simulink model "LevitadorMagnetico_act3"  (R2021a)
settings: Solver=ode1  StartTime=0.0  StopTime=1  FixedStep=0.001  RelTol=1e-3
settings Model: Creator=zeta  LastModifiedBy=zeta

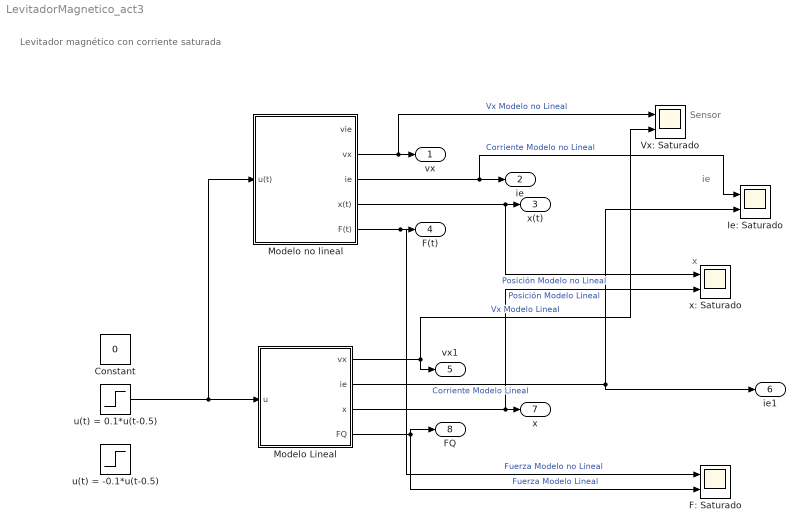
== system LevitadorMagnetico_act3 ==
  note: Levitador magnético con corriente saturada
  note: ie
  note: Sensor
  note: x
  Constant : Constant  Value=0
  F: Saturado : Scope  NumInputPorts=2
  Ie: Saturado : Scope  NumInputPorts=2
  Modelo Lineal : Subsystem  mask{Ka=3, Km=1, K1=5888, K2=1536, R=20, L=0.2, uQ=0, xQ=3.2, vxQ=3.2, ieQ=0, vx_sat_sup=0-3.2, vx_sat_inf=-10-3.2, x_sat_sup=10-3.2, x_sat_inf=-3.2, m=0.15, g=1000}
      mask prompts: vx_sat_sup "(vx_sat_sup - vxQ)"; vx_sat_inf "(vx_sat_inf- vxQ)"; x_sat_sup "(x_sat_sup - xQ)"; x_sat_inf "(x_sat_inf  - xQ)"
      mask DialogControl Control2 Prompt: Punto de operación:
      mask DialogControl Control3 Prompt: Saturación:
      mask DialogControl Control4 Prompt: otros
  Modelo no lineal : Subsystem
  Vx: Saturado : Scope  NumInputPorts=2
  u(t) = -0.1*u(t-0.5) : Step  Time=0.5  After=-0.1  SampleTime=0
  u(t) = 0.1*u(t-0.5) : Step  Time=0.5  After=0.1  SampleTime=0
  x: Saturado : Scope  NumInputPorts=2
  vx : Outport
  ie : Outport  Port=2
  x(t) : Outport  Port=3
  F(t) : Outport  Port=4
  vx1 : Outport  Port=5
  ie1 : Outport  Port=6
  x : Outport  Port=7
  FQ : Outport  Port=8
  wires:
  Modelo no lineal/2(vx) -> Vx: Saturado/1, vx/1  "Vx Modelo no Lineal"
  Modelo no lineal/4(x(t)) -> x: Saturado/1, x(t)/1  "Posición Modelo no Lineal"
  Modelo no lineal/5(F(t)) -> F: Saturado/1, F(t)/1  "Fuerza Modelo no Lineal"
  Modelo Lineal/4(FQ) -> F: Saturado/2, FQ/1  "Fuerza Modelo Lineal"
  Modelo Lineal/2(ie) -> ie1/1, Ie: Saturado/2  "Corriente Modelo Lineal"
  Modelo Lineal/1(vx) -> vx1/1, Vx: Saturado/2  "Vx Modelo Lineal"
  Modelo Lineal/3(x) -> x: Saturado/2, x/1  "Posición Modelo Lineal"
  Modelo no lineal/3(ie) -> Ie: Saturado/1, ie/1  "Corriente Modelo no Lineal"
  u(t) = 0.1*u(t-0.5)/1 -> Modelo no lineal/1(u(t)), Modelo Lineal/1(u)

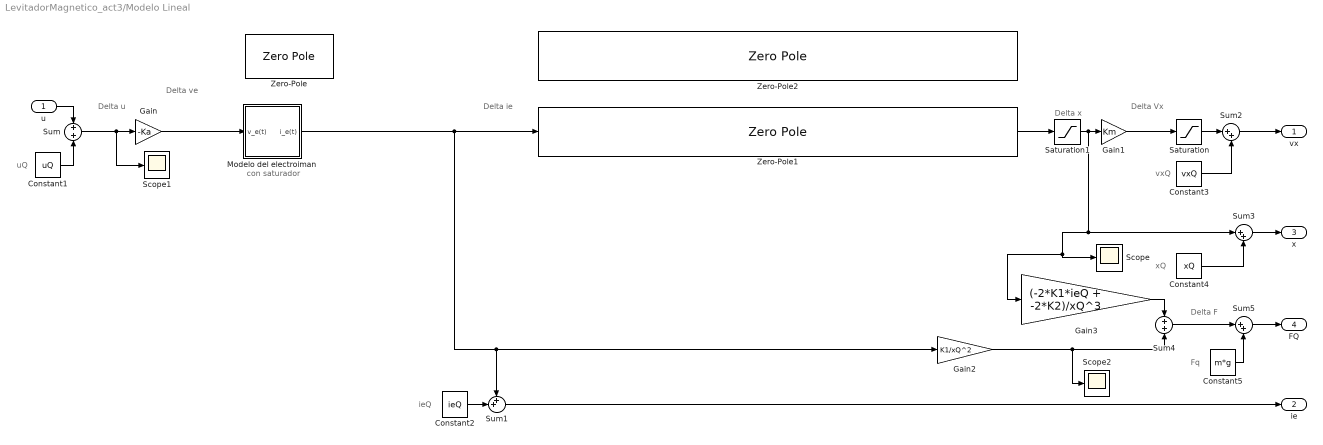
== system LevitadorMagnetico_act3/Modelo Lineal ==
  note: con saturador
  note: Fq
  note: Delta F
  note: vxQ
  note: Delta Vx
  note: Delta x
  note: Delta ie
  note: Delta ve
  note: Delta u
  note: uQ
  note: ieQ
  note: xQ
  u : Inport
  Constant1 : Constant  Value=uQ
  Constant2 : Constant  Value=ieQ
  Constant3 : Constant  Value=vxQ
  Constant4 : Constant  Value=xQ
  Constant5 : Constant  Value=m*g
  Gain : Gain  Gain=-Ka
  Gain1 : Gain  Gain=Km
  Gain2 : Gain  Gain=K1/xQ^2
  Gain3 : Gain  Gain=(-2*K1*ieQ + -2*K2)/xQ^3
  Modelo del electroiman : Subsystem  mask{L=0.2, R=20, ve_0=0}
      mask prompts: L "L [H]"; R "R [ohm]"; ve_0 "ve_0 [V]"
  Saturation : Saturate  UpperLimit=vx_sat_sup  LowerLimit=vx_sat_inf
  Saturation1 : Saturate  UpperLimit=x_sat_sup  LowerLimit=x_sat_inf
  Scope : Scope
  Scope1 : Scope
  Scope2 : Scope
  Sum : Sum  Inputs=+|+
  Sum1 : Sum  Inputs=++|
  Sum2 : Sum  Inputs=|++
  Sum3 : Sum  Inputs=|++
  Sum4 : Sum  Inputs=+|+
  Sum5 : Sum  Inputs=|++
  Zero-Pole : ZeroPole  Zeros=[]  Poles=[-R/L]  Gain=[1/L]
  Zero-Pole1 : ZeroPole  Zeros=[]  Poles=[-25 25]  Gain=[-K1/(m*xQ^2) ]
  Zero-Pole2 : ZeroPole  Zeros=[]  Poles=[-sqrt(2*(K1*ieQ + K2)/(m*xQ^3)) sqrt(2*(K1*ieQ + K2)/(m*xQ^3)) ]  Gain=[-K1/ (m*xQ^2) ]
  vx : Outport
  ie : Outport  Port=2
  x : Outport  Port=3
  FQ : Outport  Port=4
  wires:
  u/1 -> Sum/1
  Sum1/1 -> ie/1
  Sum3/1 -> x/1
  Constant2/1 -> Sum1/2
  Constant4/1 -> Sum3/2
  Sum2/1 -> vx/1
  Sum4/1 -> Sum5/1
  Gain1/1 -> Saturation/1
  Saturation/1 -> Sum2/1
  Zero-Pole1/1 -> Saturation1/1
  Constant5/1 -> Sum5/2
  Modelo del electroiman/1(i_e(t)) -> Zero-Pole1/1, Gain2/1, Sum1/1
  Saturation1/1 -> Gain1/1, Sum3/1, Scope/1, Gain3/1
  Sum5/1 -> FQ/1
  Constant1/1 -> Sum/2
  Sum/1 -> Scope1/1, Gain/1
  Constant3/1 -> Sum2/2
  Gain2/1 -> Scope2/1, Sum4/2
  Gain3/1 -> Sum4/1
  Gain/1 -> Modelo del electroiman/1(v_e(t))

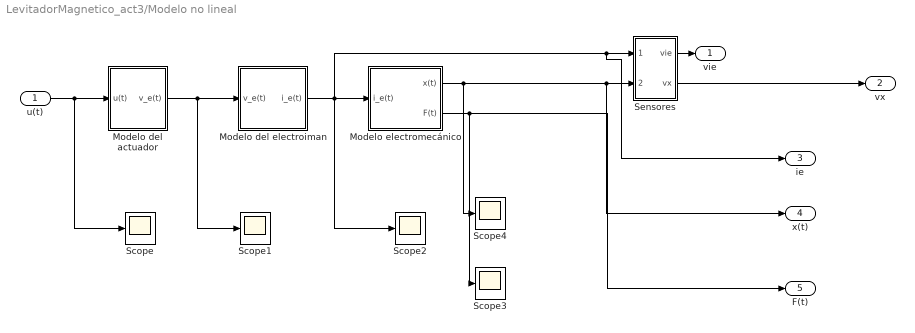
== system LevitadorMagnetico_act3/Modelo no lineal ==
  u(t) : Inport
  Modelo del actuador : Subsystem  mask{delta_a=0, K_a=3}
  Modelo del electroiman : Subsystem  mask{L=0.2, R=20, ve_0=0}
      mask prompts: L "L [H]"; R "R [ohm]"; ve_0 "ve_0 [V]"
  Modelo electromecánico : Subsystem  mask{K_1=5888, K_2=1536, m=0.15, g=1000, x0=3.2, v0=0}
  Scope{,1..4} (5 alike) : Scope
  Sensores : Subsystem  mask{delta_L=0, K_L=20/3, K_m=0, delta_m=10}
      mask prompts: K_m "1"
  vie : Outport
  vx : Outport  Port=2
  ie : Outport  Port=3
  x(t) : Outport  Port=4
  F(t) : Outport  Port=5
  wires:
  u(t)/1 -> Scope/1, Modelo del actuador/1(u(t))
  Modelo del actuador/1(v_e(t)) -> Scope1/1, Modelo del electroiman/1(v_e(t))
  Sensores/1(vie) -> vie/1
  Modelo del electroiman/1(i_e(t)) -> ie/1, Sensores/1(ie(t)), Modelo electromecánico/1(i_e(t)), Scope2/1
  Modelo electromecánico/1(x(t)) -> x(t)/1, Sensores/2(x(t)), Scope4/1
  Modelo electromecánico/2(F(t)) -> Scope3/1, F(t)/1
  Sensores/2(vx) -> vx/1

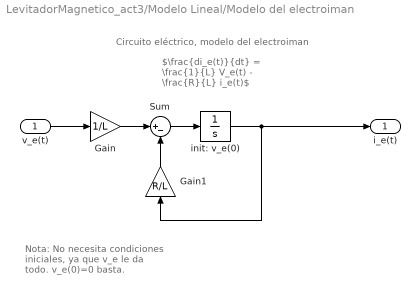
== system LevitadorMagnetico_act3/Modelo Lineal/Modelo del electroiman ==
  note: Nota: No necesita condiciones iniciales, ya que v_e le da todo.
      | v_e(0)=0 basta.
  note: $\frac{di_e(t)}{dt} = \frac{1}{L} V_e(t) - \frac{R}{L} i_e(t)$
  note: Circuito eléctrico, modelo del electroiman
  v_e(t) : Inport
  Gain : Gain  Gain=1/L
  Gain1 : Gain  Gain=R/L
  Sum : Sum  Inputs=|+-
  init: v_e(0) : Integrator  InitialCondition=ve_0  LimitOutput=on  UpperSaturationLimit=0.01  LowerSaturationLimit=-0.01
  i_e(t) : Outport
  wires:
  v_e(t)/1 -> Gain/1
  Gain/1 -> Sum/1
  init: v_e(0)/1 -> i_e(t)/1, Gain1/1
  Gain1/1 -> Sum/2
  Sum/1 -> init: v_e(0)/1

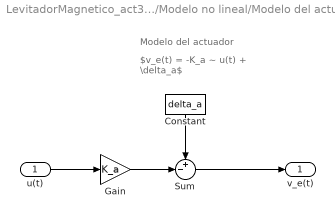
== system LevitadorMagnetico_act3/Modelo no lineal/Modelo del actuador ==
  note: $v_e(t) = -K_a ~ u(t) + \delta_a$
  note: Modelo del actuador
  u(t) : Inport
  Constant : Constant  Value=delta_a
  Gain : Gain  Gain=K_a
  Sum : Sum  Inputs=+-|
  v_e(t) : Outport
  wires:
  Constant/1 -> Sum/1
  Gain/1 -> Sum/2
  Sum/1 -> v_e(t)/1
  u(t)/1 -> Gain/1

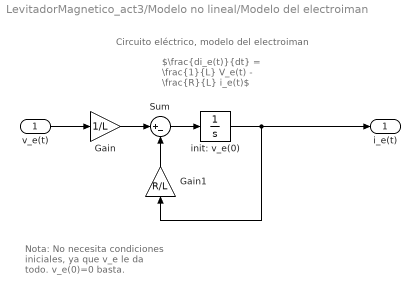
== system LevitadorMagnetico_act3/Modelo no lineal/Modelo del electroiman ==
  note: Nota: No necesita condiciones iniciales, ya que v_e le da todo.
      | v_e(0)=0 basta.
  note: $\frac{di_e(t)}{dt} = \frac{1}{L} V_e(t) - \frac{R}{L} i_e(t)$
  note: Circuito eléctrico, modelo del electroiman
  v_e(t) : Inport
  Gain : Gain  Gain=1/L
  Gain1 : Gain  Gain=R/L
  Sum : Sum  Inputs=|+-
  init: v_e(0) : Integrator  InitialCondition=ve_0  LimitOutput=on  UpperSaturationLimit=0.01  LowerSaturationLimit=-0.01
  i_e(t) : Outport
  wires:
  v_e(t)/1 -> Gain/1
  Gain/1 -> Sum/1
  init: v_e(0)/1 -> i_e(t)/1, Gain1/1
  Gain1/1 -> Sum/2
  Sum/1 -> init: v_e(0)/1

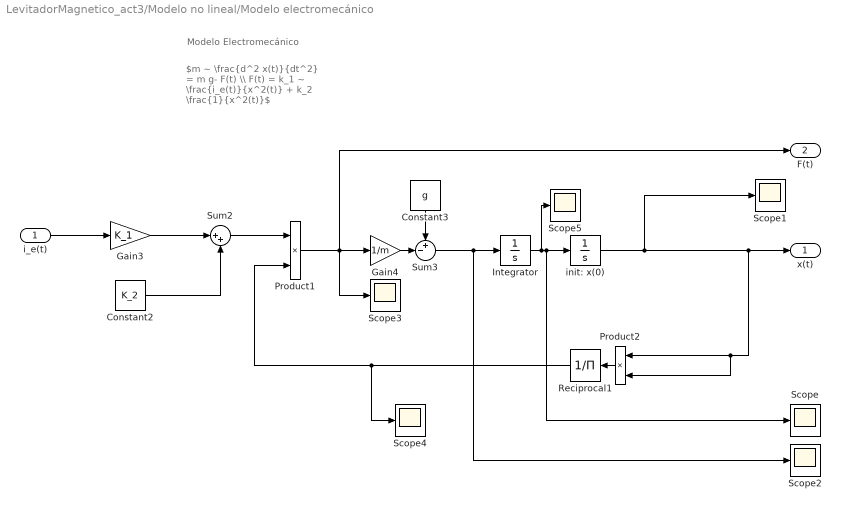
== system LevitadorMagnetico_act3/Modelo no lineal/Modelo electromecánico ==
  note: $m ~ \frac{d^2 x(t)}{dt^2} = m g- F(t) \\ F(t) = k_1 ~ \frac{i_e(t)}{x^2(t)} + k_2 \frac{1}{x^2(t)}$
  note: Modelo Electromecánico
  i_e(t) : Inport
  Constant2 : Constant  Value=K_2
  Constant3 : Constant  Value=g
  Gain3 : Gain  Gain=K_1
  Gain4 : Gain  Gain=1/m
  Integrator : Integrator  InitialCondition=v0  LowerSaturationLimit=0
  Product1 : Product
  Product2 : Product
  Reciprocal1 : Product  Inputs=/
  Scope{,1..5} (6 alike) : Scope
  Sum2 : Sum  Inputs=|++
  Sum3 : Sum  Inputs=+-|
  init: x(0) : Integrator  InitialCondition=x0  LimitOutput=on  UpperSaturationLimit=10  LowerSaturationLimit=1e-10
  x(t) : Outport
  F(t) : Outport  Port=2
  wires:
  i_e(t)/1 -> Gain3/1
  Gain3/1 -> Sum2/1
  Constant2/1 -> Sum2/2
  Sum2/1 -> Product1/1
  Constant3/1 -> Sum3/1
  Gain4/1 -> Sum3/2
  Sum3/1 -> Scope2/1, Integrator/1
  Product2/1 -> Reciprocal1/1
  init: x(0)/1 -> x(t)/1, Product2/1, Product2/2, Scope1/1
  Reciprocal1/1 -> Scope4/1, Product1/2
  Integrator/1 -> Scope5/1, init: x(0)/1, Scope/1
  Product1/1 -> Scope3/1, F(t)/1, Gain4/1

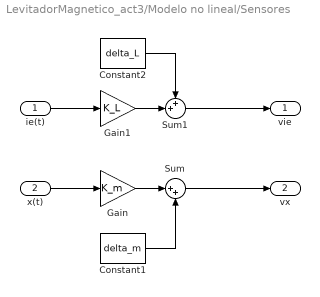
== system LevitadorMagnetico_act3/Modelo no lineal/Sensores ==
  ie(t) : Inport
  x(t) : Inport  Port=2
  Constant1 : Constant  Value=delta_m
  Constant2 : Constant  Value=delta_L
  Gain : Gain  Gain=K_m
  Gain1 : Gain  Gain=K_L
  Sum : Sum  Inputs=|++
  Sum1 : Sum  Inputs=++|
  vie : Outport
  vx : Outport  Port=2
  wires:
  Gain1/1 -> Sum1/2
  Gain/1 -> Sum/1
  Sum1/1 -> vie/1
  Constant2/1 -> Sum1/1
  Sum/1 -> vx/1
  Constant1/1 -> Sum/2
  ie(t)/1 -> Gain1/1
  x(t)/1 -> Gain/1
